simulink model "gm_uz_pmsm_model_9ph_dq"  (R2021b)
settings: Solver=FixedStepAuto  StartTime=0.0  StopTime=0.8  RelTol=1e-3
undefined symbols (not defined in the file or in its folder): c, friction_coefficient, inertia, k_i_d, k_i_q, k_p_d, k_p_q, Kpd, L_d, L_q, L_x1, L_x2, L_x3, L_y1, L_y2, L_y3, L_zero, polepair, psi_pm, R_1, static_friction_torque, Tnd
libraries: hdlmdlgenlib x137, dspsigops x19, slpidlib x2, pid_lib x1, spsdq0toAlphaBetaZeroLib x1
(part 2 of 2)

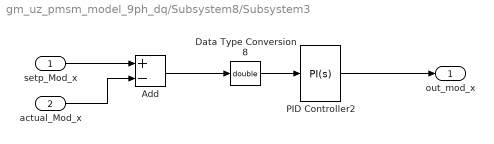
== system gm_uz_pmsm_model_9ph_dq/Subsystem8/Subsystem3 ==
  setp_Mod_x : Inport
  actual_Mod_x : Inport  Port=2
  Add : Sum  Inputs=+-
  Data Type Conversion8 : DataTypeConversion  OutDataTypeStr=double
  PID Controller2 : slpidlib/PID Controller  Controller=PI  Form=Ideal  TimeDomain=Continuous-time  UseExternalTs=off  SampleTime=-1  IntegratorMethod=Forward Euler  FilterMethod=Forward Euler  ControllerParametersSource=internal  P=k_p_q  I=k_i_q  D=0  UseFilter=on  N=100  TunerSelectOption=Transfer Function Based (PID Tuner App)  InitialConditionSource=internal  InitialConditionForIntegrator=0  InitialConditionForFilter=0  DifferentiatorICPrevScaledInput=0  ExternalReset=none  TrackingMode=off  Kt=1  LimitOutput=on  SatLimitsSource=internal  UpperSaturationLimit=100  LowerSaturationLimit=-100  LinearizeAsGain=on  AntiWindupMode=clamping  Kb=1  POutMin=[]  POutMax=[]  IOutMin=[]  IOutMax=[]  DOutMin=[]  DOutMax=[]  NOutMin=[]  NOutMax=[]  SumOutMin=[]  SumOutMax=[]  SaturationOutMin=[]  SaturationOutMax=[]  PParamMin=[]  PParamMax=[]  IParamMin=[]  IParamMax=[]  DParamMin=[]  DParamMax=[]  NParamMin=[]  NParamMax=[]  KbParamMin=[]  KbParamMax=[]  KtParamMin=[]  KtParamMax=[]  KbOutMin=[]  KbOutMax=[]  KtOutMin=[]  KtOutMax=[]  IntegratorOutMin=[]  IntegratorOutMax=[]  FilterOutMin=[]  FilterOutMax=[]  SumI1OutMin=[]  SumI1OutMax=[]  SumI2OutMin=[]  SumI2OutMax=[]  SumI3OutMin=[]  SumI3OutMax=[]  SumI4OutMin=[]  SumI4OutMax=[]  SumDOutMin=[]  SumDOutMax=[]  DifferentiatorOutMin=[]  DifferentiatorOutMax=[]  FilterDiffOutCoefMin=[]  FilterDiffOutCoefMax=[]  ReciprocalOutMin=[]  ReciprocalOutMax=[]  SumDenOutMin=[]  SumDenOutMax=[]  SumNumOutMin=[]  SumNumOutMax=[]  DivideOutMin=[]  DivideOutMax=[]  UdiffTsProdOutMin=[]  UdiffTsProdOutMax=[]  NTsProdOutMin=[]  NTsProdOutMax=[]  UintegralTsProdOutMin=[]  UintegralTsProdOutMax=[]  UngainTsProdOutMin=[]  UngainTsProdOutMax=[]  IntegratorContinuousStateAttributes=''  IntegratorStateMustResolveToSignalObject=off  IntegratorRTWStateStorageClass=Auto  FilterContinuousStateAttributes=''  FilterStateMustResolveToSignalObject=off  FilterRTWStateStorageClass=Auto  ParallelPVariant=Passthrough  IdealPVariant=InternalParameters  IVariant=InternalParameters  DVariant=Disabled  IntegratorVariant=Continuous  SatVariant=Enabled  AWVariant=ContClampingIdeal  PCopyVariant=InternalParamsIdeal  TRVariant=Disabled  FdbkBlocksVariant=Forward  IdealPFdbkVariant=Disabled  SatFdbkVariant=Disabled  DerivativeFilterVariant=Disabled  NVariant=Disabled  NCopyVariant=Disabled_SignalSpec  FilterICVariant=Disabled  IntegratorICVariant=InternalICs  ExternalResetVariant=Disabled  TRSumVariant=Passthrough  SumFdbkVariant=Disabled  SumVariant=Sum_PI  TsampFilterVariant=InternalTs  TsampNgainVariant=Passthrough  TsampIntegralVariant=Passthrough  ExternalSaturationOutDataTypeStr=Inherit: Same as second input
  out_mod_x : Outport
  wires:
  Add/1 -> Data Type Conversion8/1
  actual_Mod_x/1 -> Add/2
  Data Type Conversion8/1 -> PID Controller2/1
  setp_Mod_x/1 -> Add/1
  PID Controller2/1 -> out_mod_x/1

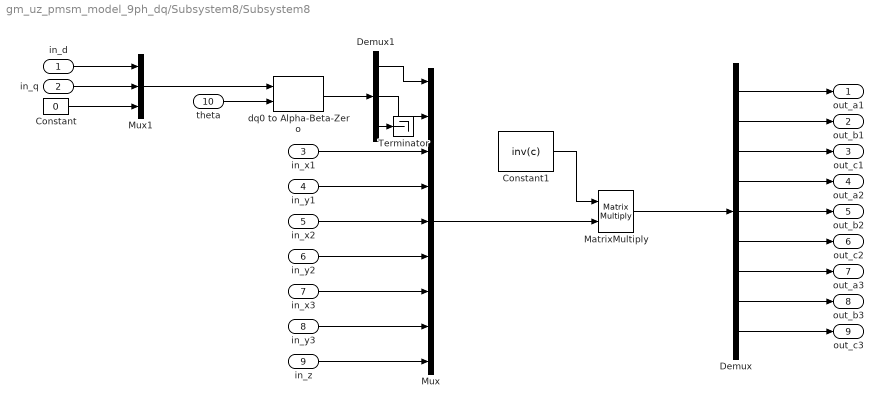
== system gm_uz_pmsm_model_9ph_dq/Subsystem8/Subsystem8 ==
  in_d : Inport
  in_q : Inport  Port=2
  in_x1 : Inport  Port=3
  in_y1 : Inport  Port=4
  in_x2 : Inport  Port=5
  in_y2 : Inport  Port=6
  in_x3 : Inport  Port=7
  in_y3 : Inport  Port=8
  in_z : Inport  Port=9
  theta : Inport  Port=10
  Constant : Constant  Value=0  SampleTime=-1
  Constant1 : Constant  Value=inv(c)
  Demux : Demux  Outputs=9
  Demux1 : Demux  Outputs=3
  MatrixMultiply : Product  Multiplication=Matrix(*)
  Mux : Mux  Inputs=9
  Mux1 : Mux  Inputs=3
  Terminator : Terminator
  dq0 to Alpha-Beta-Zero : spsdq0toAlphaBetaZeroLib/dq0 to Alpha-Beta-Zero  Alignment=90 degrees behind phase A axis
      settings: SourceProductBaseCode=PS
  out_a1 : Outport
  out_b1 : Outport  Port=2
  out_c1 : Outport  Port=3
  out_a2 : Outport  Port=4
  out_b2 : Outport  Port=5
  out_c2 : Outport  Port=6
  out_a3 : Outport  Port=7
  out_b3 : Outport  Port=8
  out_c3 : Outport  Port=9
  wires:
  Demux/7 -> out_a3/1
  Demux/9 -> out_c3/1
  Demux/8 -> out_b3/1
  Demux/5 -> out_b2/1
  Demux/6 -> out_c2/1
  Demux/4 -> out_a2/1
  Demux/3 -> out_c1/1
  Demux/2 -> out_b1/1
  Constant1/1 -> MatrixMultiply/1
  Demux1/3 -> Terminator/1
  Demux1/2 -> Mux/2
  Demux1/1 -> Mux/1
  dq0 to Alpha-Beta-Zero/1 -> Demux1/1
  theta/1 -> dq0 to Alpha-Beta-Zero/2
  Mux1/1 -> dq0 to Alpha-Beta-Zero/1
  in_d/1 -> Mux1/1
  in_q/1 -> Mux1/2
  Constant/1 -> Mux1/3
  in_z/1 -> Mux/9
  in_x2/1 -> Mux/5
  Mux/1 -> MatrixMultiply/2
  in_y1/1 -> Mux/4
  in_x1/1 -> Mux/3
  Demux/1 -> out_a1/1
  in_y2/1 -> Mux/6
  MatrixMultiply/1 -> Demux/1
  in_y3/1 -> Mux/8
  in_x3/1 -> Mux/7

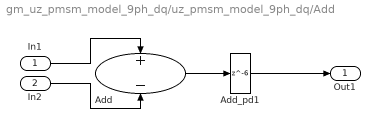
== system gm_uz_pmsm_model_9ph_dq/uz_pmsm_model_9ph_dq/Add ==
  In1 : Inport
  In2 : Inport  Port=2
  Add : Sum  Inputs=+-  OutDataTypeStr=double  SampleTime=1e-08
  Add_pd1 : Delay  DelayLength=6
  Out1 : Outport
  wires:
  In1/1 -> Add/1
  In2/1 -> Add/2
  Add/1 -> Add_pd1/1
  Add_pd1/1 -> Out1/1

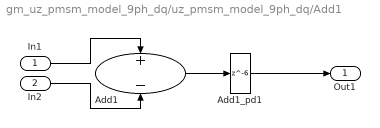
== system gm_uz_pmsm_model_9ph_dq/uz_pmsm_model_9ph_dq/Add1 ==
  In1 : Inport
  In2 : Inport  Port=2
  Add1 : Sum  Inputs=+-  OutDataTypeStr=double  SampleTime=1e-08
  Add1_pd1 : Delay  DelayLength=6
  Out1 : Outport
  wires:
  In1/1 -> Add1/1
  In2/1 -> Add1/2
  Add1/1 -> Add1_pd1/1
  Add1_pd1/1 -> Out1/1

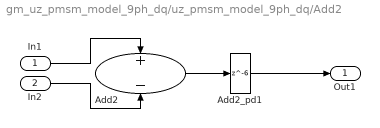
== system gm_uz_pmsm_model_9ph_dq/uz_pmsm_model_9ph_dq/Add2 ==
  In1 : Inport
  In2 : Inport  Port=2
  Add2 : Sum  Inputs=+-  OutDataTypeStr=double  SampleTime=1e-08
  Add2_pd1 : Delay  DelayLength=6
  Out1 : Outport
  wires:
  In1/1 -> Add2/1
  In2/1 -> Add2/2
  Add2/1 -> Add2_pd1/1
  Add2_pd1/1 -> Out1/1

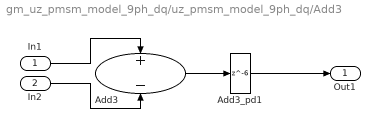
== system gm_uz_pmsm_model_9ph_dq/uz_pmsm_model_9ph_dq/Add3 ==
  In1 : Inport
  In2 : Inport  Port=2
  Add3 : Sum  Inputs=+-  OutDataTypeStr=double  SampleTime=1e-08
  Add3_pd1 : Delay  DelayLength=6
  Out1 : Outport
  wires:
  In1/1 -> Add3/1
  In2/1 -> Add3/2
  Add3/1 -> Add3_pd1/1
  Add3_pd1/1 -> Out1/1

== system gm_uz_pmsm_model_9ph_dq/uz_pmsm_model_9ph_dq/Add4 ==
  In1 : Inport
  In2 : Inport  Port=2
  Add4 : Sum  Inputs=+-  OutDataTypeStr=double  SampleTime=1e-08
  Add4_pd1 : Delay  DelayLength=6
  Out1 : Outport
  wires:
  In1/1 -> Add4/1
  In2/1 -> Add4/2
  Add4/1 -> Add4_pd1/1
  Add4_pd1/1 -> Out1/1

== system gm_uz_pmsm_model_9ph_dq/uz_pmsm_model_9ph_dq/Add5 ==
  In1 : Inport
  In2 : Inport  Port=2
  Add5 : Sum  Inputs=+-  OutDataTypeStr=double  SampleTime=1e-08
  Add5_pd1 : Delay  DelayLength=6
  Out1 : Outport
  wires:
  In1/1 -> Add5/1
  In2/1 -> Add5/2
  Add5/1 -> Add5_pd1/1
  Add5_pd1/1 -> Out1/1

== system gm_uz_pmsm_model_9ph_dq/uz_pmsm_model_9ph_dq/Add6 ==
  In1 : Inport
  In2 : Inport  Port=2
  Add6 : Sum  Inputs=+-  OutDataTypeStr=double  SampleTime=1e-08
  Add6_pd1 : Delay  DelayLength=6
  Out1 : Outport
  wires:
  In1/1 -> Add6/1
  In2/1 -> Add6/2
  Add6/1 -> Add6_pd1/1
  Add6_pd1/1 -> Out1/1

== system gm_uz_pmsm_model_9ph_dq/uz_pmsm_model_9ph_dq/Compare To Constant1_relop ==
  In1 : Inport
  In2 : Inport  Port=2
  Compare To Constant1_relop : RelationalOperator  Operator=<  OutDataTypeStr=boolean  SampleTime=1e-08  RndMeth=Nearest  InputSameDT=on
  Compare To Constant1_relop_pd1 : Delay  DelayLength=1
  Out1 : Outport
  wires:
  In1/1 -> Compare To Constant1_relop/1
  In2/1 -> Compare To Constant1_relop/2
  Compare To Constant1_relop/1 -> Compare To Constant1_relop_pd1/1
  Compare To Constant1_relop_pd1/1 -> Out1/1

== system gm_uz_pmsm_model_9ph_dq/uz_pmsm_model_9ph_dq/Compare To Constant_relop ==
  In1 : Inport
  In2 : Inport  Port=2
  Compare To Constant_relop : RelationalOperator  OutDataTypeStr=boolean  SampleTime=1e-08  RndMeth=Nearest  InputSameDT=on
  Compare To Constant_relop_pd1 : Delay  DelayLength=1
  Out1 : Outport
  wires:
  In1/1 -> Compare To Constant_relop/1
  In2/1 -> Compare To Constant_relop/2
  Compare To Constant_relop/1 -> Compare To Constant_relop_pd1/1
  Compare To Constant_relop_pd1/1 -> Out1/1

== system gm_uz_pmsm_model_9ph_dq/uz_pmsm_model_9ph_dq/Data Type Conversion1 ==
  In1 : Inport
  Data Type Conversion1 : DataTypeConversion  OutDataTypeStr=double  RndMeth=Nearest  SampleTime=1e-08
  Data Type Conversion1_pd1 : Delay  DelayLength=3
  Out1 : Outport
  wires:
  In1/1 -> Data Type Conversion1/1
  Data Type Conversion1/1 -> Data Type Conversion1_pd1/1
  Data Type Conversion1_pd1/1 -> Out1/1

== system gm_uz_pmsm_model_9ph_dq/uz_pmsm_model_9ph_dq/Data Type Conversion10 ==
  In1 : Inport
  Data Type Conversion10 : DataTypeConversion  OutDataTypeStr=double  RndMeth=Nearest  SampleTime=1e-08
  Data Type Conversion10_pd1 : Delay  DelayLength=3
  Out1 : Outport
  wires:
  In1/1 -> Data Type Conversion10/1
  Data Type Conversion10/1 -> Data Type Conversion10_pd1/1
  Data Type Conversion10_pd1/1 -> Out1/1

== system gm_uz_pmsm_model_9ph_dq/uz_pmsm_model_9ph_dq/Data Type Conversion101 ==
  In1 : Inport
  Data Type Conversion101 : DataTypeConversion  OutDataTypeStr=double  RndMeth=Nearest  SampleTime=1e-08
  Data Type Conversion101_pd1 : Delay  DelayLength=3
  Out1 : Outport
  wires:
  In1/1 -> Data Type Conversion101/1
  Data Type Conversion101/1 -> Data Type Conversion101_pd1/1
  Data Type Conversion101_pd1/1 -> Out1/1

== system gm_uz_pmsm_model_9ph_dq/uz_pmsm_model_9ph_dq/Data Type Conversion11 ==
  In1 : Inport
  Data Type Conversion11 : DataTypeConversion  OutDataTypeStr=single  RndMeth=Nearest  SampleTime=1e-08
  Data Type Conversion11_pd1 : Delay  DelayLength=3
  Out1 : Outport
  wires:
  In1/1 -> Data Type Conversion11/1
  Data Type Conversion11/1 -> Data Type Conversion11_pd1/1
  Data Type Conversion11_pd1/1 -> Out1/1

== system gm_uz_pmsm_model_9ph_dq/uz_pmsm_model_9ph_dq/Data Type Conversion111 ==
  In1 : Inport
  Data Type Conversion111 : DataTypeConversion  OutDataTypeStr=double  RndMeth=Nearest  SampleTime=1e-08
  Data Type Conversion111_pd1 : Delay  DelayLength=3
  Out1 : Outport
  wires:
  In1/1 -> Data Type Conversion111/1
  Data Type Conversion111/1 -> Data Type Conversion111_pd1/1
  Data Type Conversion111_pd1/1 -> Out1/1

== system gm_uz_pmsm_model_9ph_dq/uz_pmsm_model_9ph_dq/Data Type Conversion12 ==
  In1 : Inport
  Data Type Conversion12 : DataTypeConversion  OutDataTypeStr=fixdt(1, 18, 14)  RndMeth=Nearest  SampleTime=1e-08
  Data Type Conversion12_pd1 : Delay  DelayLength=3
  Out1 : Outport
  wires:
  In1/1 -> Data Type Conversion12/1
  Data Type Conversion12/1 -> Data Type Conversion12_pd1/1
  Data Type Conversion12_pd1/1 -> Out1/1

== system gm_uz_pmsm_model_9ph_dq/uz_pmsm_model_9ph_dq/Data Type Conversion121 ==
  In1 : Inport
  Data Type Conversion121 : DataTypeConversion  OutDataTypeStr=double  RndMeth=Nearest  SampleTime=1e-08
  Data Type Conversion121_pd1 : Delay  DelayLength=3
  Out1 : Outport
  wires:
  In1/1 -> Data Type Conversion121/1
  Data Type Conversion121/1 -> Data Type Conversion121_pd1/1
  Data Type Conversion121_pd1/1 -> Out1/1

== system gm_uz_pmsm_model_9ph_dq/uz_pmsm_model_9ph_dq/Data Type Conversion13 ==
  In1 : Inport
  Data Type Conversion13 : DataTypeConversion  OutDataTypeStr=double  RndMeth=Nearest  SampleTime=1e-08
  Data Type Conversion13_pd1 : Delay  DelayLength=3
  Out1 : Outport
  wires:
  In1/1 -> Data Type Conversion13/1
  Data Type Conversion13/1 -> Data Type Conversion13_pd1/1
  Data Type Conversion13_pd1/1 -> Out1/1

== system gm_uz_pmsm_model_9ph_dq/uz_pmsm_model_9ph_dq/Data Type Conversion14 ==
  In1 : Inport
  Data Type Conversion14 : DataTypeConversion  OutDataTypeStr=single  RndMeth=Nearest  SampleTime=1e-08
  Data Type Conversion14_pd1 : Delay  DelayLength=3
  Out1 : Outport
  wires:
  In1/1 -> Data Type Conversion14/1
  Data Type Conversion14/1 -> Data Type Conversion14_pd1/1
  Data Type Conversion14_pd1/1 -> Out1/1

== system gm_uz_pmsm_model_9ph_dq/uz_pmsm_model_9ph_dq/Data Type Conversion15 ==
  In1 : Inport
  Data Type Conversion15 : DataTypeConversion  OutDataTypeStr=double  RndMeth=Nearest  SampleTime=1e-08
  Data Type Conversion15_pd1 : Delay  DelayLength=3
  Out1 : Outport
  wires:
  In1/1 -> Data Type Conversion15/1
  Data Type Conversion15/1 -> Data Type Conversion15_pd1/1
  Data Type Conversion15_pd1/1 -> Out1/1

== system gm_uz_pmsm_model_9ph_dq/uz_pmsm_model_9ph_dq/Data Type Conversion2 ==
  In1 : Inport
  Data Type Conversion2 : DataTypeConversion  OutDataTypeStr=double  RndMeth=Nearest  SampleTime=1e-08
  Data Type Conversion2_pd1 : Delay  DelayLength=3
  Out1 : Outport
  wires:
  In1/1 -> Data Type Conversion2/1
  Data Type Conversion2/1 -> Data Type Conversion2_pd1/1
  Data Type Conversion2_pd1/1 -> Out1/1

== system gm_uz_pmsm_model_9ph_dq/uz_pmsm_model_9ph_dq/Data Type Conversion21 ==
  In1 : Inport
  Data Type Conversion21 : DataTypeConversion  OutDataTypeStr=double  RndMeth=Nearest  SampleTime=1e-08
  Data Type Conversion21_pd1 : Delay  DelayLength=3
  Out1 : Outport
  wires:
  In1/1 -> Data Type Conversion21/1
  Data Type Conversion21/1 -> Data Type Conversion21_pd1/1
  Data Type Conversion21_pd1/1 -> Out1/1

== system gm_uz_pmsm_model_9ph_dq/uz_pmsm_model_9ph_dq/Data Type Conversion3 ==
  In1 : Inport
  Data Type Conversion3 : DataTypeConversion  OutDataTypeStr=fixdt(1, 27, 18)  RndMeth=Nearest  SampleTime=1e-08
  Data Type Conversion3_pd1 : Delay  DelayLength=3
  Out1 : Outport
  wires:
  In1/1 -> Data Type Conversion3/1
  Data Type Conversion3/1 -> Data Type Conversion3_pd1/1
  Data Type Conversion3_pd1/1 -> Out1/1

== system gm_uz_pmsm_model_9ph_dq/uz_pmsm_model_9ph_dq/Data Type Conversion31 ==
  In1 : Inport
  Data Type Conversion31 : DataTypeConversion  OutDataTypeStr=double  RndMeth=Nearest  SampleTime=1e-08
  Data Type Conversion31_pd1 : Delay  DelayLength=3
  Out1 : Outport
  wires:
  In1/1 -> Data Type Conversion31/1
  Data Type Conversion31/1 -> Data Type Conversion31_pd1/1
  Data Type Conversion31_pd1/1 -> Out1/1

== system gm_uz_pmsm_model_9ph_dq/uz_pmsm_model_9ph_dq/Data Type Conversion4 ==
  In1 : Inport
  Data Type Conversion4 : DataTypeConversion  OutDataTypeStr=single  RndMeth=Nearest  SampleTime=1e-08
  Data Type Conversion4_pd1 : Delay  DelayLength=3
  Out1 : Outport
  wires:
  In1/1 -> Data Type Conversion4/1
  Data Type Conversion4/1 -> Data Type Conversion4_pd1/1
  Data Type Conversion4_pd1/1 -> Out1/1

== system gm_uz_pmsm_model_9ph_dq/uz_pmsm_model_9ph_dq/Data Type Conversion41 ==
  In1 : Inport
  Data Type Conversion41 : DataTypeConversion  OutDataTypeStr=double  RndMeth=Nearest  SampleTime=1e-08
  Data Type Conversion41_pd1 : Delay  DelayLength=3
  Out1 : Outport
  wires:
  In1/1 -> Data Type Conversion41/1
  Data Type Conversion41/1 -> Data Type Conversion41_pd1/1
  Data Type Conversion41_pd1/1 -> Out1/1

== system gm_uz_pmsm_model_9ph_dq/uz_pmsm_model_9ph_dq/Data Type Conversion5 ==
  In1 : Inport
  Data Type Conversion5 : DataTypeConversion  OutDataTypeStr=single  RndMeth=Nearest  SampleTime=1e-08
  Data Type Conversion5_pd1 : Delay  DelayLength=3
  Out1 : Outport
  wires:
  In1/1 -> Data Type Conversion5/1
  Data Type Conversion5/1 -> Data Type Conversion5_pd1/1
  Data Type Conversion5_pd1/1 -> Out1/1

== system gm_uz_pmsm_model_9ph_dq/uz_pmsm_model_9ph_dq/Data Type Conversion51 ==
  In1 : Inport
  Data Type Conversion51 : DataTypeConversion  OutDataTypeStr=double  RndMeth=Nearest  SampleTime=1e-08
  Data Type Conversion51_pd1 : Delay  DelayLength=3
  Out1 : Outport
  wires:
  In1/1 -> Data Type Conversion51/1
  Data Type Conversion51/1 -> Data Type Conversion51_pd1/1
  Data Type Conversion51_pd1/1 -> Out1/1

== system gm_uz_pmsm_model_9ph_dq/uz_pmsm_model_9ph_dq/Data Type Conversion6 ==
  In1 : Inport
  Data Type Conversion6 : DataTypeConversion  OutDataTypeStr=double  RndMeth=Nearest  SampleTime=1e-08
  Data Type Conversion6_pd1 : Delay  DelayLength=3
  Out1 : Outport
  wires:
  In1/1 -> Data Type Conversion6/1
  Data Type Conversion6/1 -> Data Type Conversion6_pd1/1
  Data Type Conversion6_pd1/1 -> Out1/1

== system gm_uz_pmsm_model_9ph_dq/uz_pmsm_model_9ph_dq/Data Type Conversion61 ==
  In1 : Inport
  Data Type Conversion61 : DataTypeConversion  OutDataTypeStr=double  RndMeth=Nearest  SampleTime=1e-08
  Data Type Conversion61_pd1 : Delay  DelayLength=3
  Out1 : Outport
  wires:
  In1/1 -> Data Type Conversion61/1
  Data Type Conversion61/1 -> Data Type Conversion61_pd1/1
  Data Type Conversion61_pd1/1 -> Out1/1

== system gm_uz_pmsm_model_9ph_dq/uz_pmsm_model_9ph_dq/Data Type Conversion7 ==
  In1 : Inport
  Data Type Conversion7 : DataTypeConversion  OutDataTypeStr=double  RndMeth=Nearest  SampleTime=1e-08
  Data Type Conversion7_pd1 : Delay  DelayLength=3
  Out1 : Outport
  wires:
  In1/1 -> Data Type Conversion7/1
  Data Type Conversion7/1 -> Data Type Conversion7_pd1/1
  Data Type Conversion7_pd1/1 -> Out1/1

== system gm_uz_pmsm_model_9ph_dq/uz_pmsm_model_9ph_dq/Data Type Conversion71 ==
  In1 : Inport
  Data Type Conversion71 : DataTypeConversion  OutDataTypeStr=double  RndMeth=Nearest  SampleTime=1e-08
  Data Type Conversion71_pd1 : Delay  DelayLength=3
  Out1 : Outport
  wires:
  In1/1 -> Data Type Conversion71/1
  Data Type Conversion71/1 -> Data Type Conversion71_pd1/1
  Data Type Conversion71_pd1/1 -> Out1/1

== system gm_uz_pmsm_model_9ph_dq/uz_pmsm_model_9ph_dq/Data Type Conversion8 ==
  In1 : Inport
  Data Type Conversion8 : DataTypeConversion  OutDataTypeStr=double  RndMeth=Nearest  SampleTime=1e-08
  Data Type Conversion8_pd1 : Delay  DelayLength=3
  Out1 : Outport
  wires:
  In1/1 -> Data Type Conversion8/1
  Data Type Conversion8/1 -> Data Type Conversion8_pd1/1
  Data Type Conversion8_pd1/1 -> Out1/1

== system gm_uz_pmsm_model_9ph_dq/uz_pmsm_model_9ph_dq/Data Type Conversion81 ==
  In1 : Inport
  Data Type Conversion81 : DataTypeConversion  OutDataTypeStr=single  RndMeth=Nearest  SampleTime=1e-08
  Data Type Conversion81_pd1 : Delay  DelayLength=3
  Out1 : Outport
  wires:
  In1/1 -> Data Type Conversion81/1
  Data Type Conversion81/1 -> Data Type Conversion81_pd1/1
  Data Type Conversion81_pd1/1 -> Out1/1

== system gm_uz_pmsm_model_9ph_dq/uz_pmsm_model_9ph_dq/Data Type Conversion9 ==
  In1 : Inport
  Data Type Conversion9 : DataTypeConversion  OutDataTypeStr=double  RndMeth=Nearest  SampleTime=1e-08
  Data Type Conversion9_pd1 : Delay  DelayLength=3
  Out1 : Outport
  wires:
  In1/1 -> Data Type Conversion9/1
  Data Type Conversion9/1 -> Data Type Conversion9_pd1/1
  Data Type Conversion9_pd1/1 -> Out1/1

== system gm_uz_pmsm_model_9ph_dq/uz_pmsm_model_9ph_dq/Divide ==
  In1 : Inport
  In2 : Inport  Port=2
  Divide : Product  Inputs=**  OutDataTypeStr=double  SampleTime=1e-08
  Divide_pd1 : Delay  DelayLength=6
  Out1 : Outport
  wires:
  In1/1 -> Divide/1
  In2/1 -> Divide/2
  Divide/1 -> Divide_pd1/1
  Divide_pd1/1 -> Out1/1

== system gm_uz_pmsm_model_9ph_dq/uz_pmsm_model_9ph_dq/Divide1 ==
  In1 : Inport
  In2 : Inport  Port=2
  Divide1 : Product  Inputs=**  OutDataTypeStr=double  SampleTime=1e-08
  Divide1_pd1 : Delay  DelayLength=6
  Out1 : Outport
  wires:
  In1/1 -> Divide1/1
  In2/1 -> Divide1/2
  Divide1/1 -> Divide1_pd1/1
  Divide1_pd1/1 -> Out1/1

== system gm_uz_pmsm_model_9ph_dq/uz_pmsm_model_9ph_dq/Divide10 ==
  In1 : Inport
  In2 : Inport  Port=2
  Divide10 : Product  Inputs=**  OutDataTypeStr=double  SampleTime=1e-08
  Divide10_pd1 : Delay  DelayLength=6
  Out1 : Outport
  wires:
  In1/1 -> Divide10/1
  In2/1 -> Divide10/2
  Divide10/1 -> Divide10_pd1/1
  Divide10_pd1/1 -> Out1/1

== system gm_uz_pmsm_model_9ph_dq/uz_pmsm_model_9ph_dq/Divide11 ==
  In1 : Inport
  In2 : Inport  Port=2
  Divide11 : Product  Inputs=**  OutDataTypeStr=double  SampleTime=1e-08
  Divide11_pd1 : Delay  DelayLength=6
  Out1 : Outport
  wires:
  In1/1 -> Divide11/1
  In2/1 -> Divide11/2
  Divide11/1 -> Divide11_pd1/1
  Divide11_pd1/1 -> Out1/1

== system gm_uz_pmsm_model_9ph_dq/uz_pmsm_model_9ph_dq/Divide12 ==
  In1 : Inport
  In2 : Inport  Port=2
  Divide12 : Product  Inputs=**  OutDataTypeStr=double  SampleTime=1e-08
  Divide12_pd1 : Delay  DelayLength=6
  Out1 : Outport
  wires:
  In1/1 -> Divide12/1
  In2/1 -> Divide12/2
  Divide12/1 -> Divide12_pd1/1
  Divide12_pd1/1 -> Out1/1

== system gm_uz_pmsm_model_9ph_dq/uz_pmsm_model_9ph_dq/Divide13 ==
  In1 : Inport
  In2 : Inport  Port=2
  Divide13 : Product  Inputs=**  OutDataTypeStr=double  SampleTime=1e-08
  Divide13_pd1 : Delay  DelayLength=6
  Out1 : Outport
  wires:
  In1/1 -> Divide13/1
  In2/1 -> Divide13/2
  Divide13/1 -> Divide13_pd1/1
  Divide13_pd1/1 -> Out1/1

== system gm_uz_pmsm_model_9ph_dq/uz_pmsm_model_9ph_dq/Divide2 ==
  In1 : Inport
  In2 : Inport  Port=2
  Divide2 : Product  Inputs=**  OutDataTypeStr=double  SampleTime=1e-08
  Divide2_pd1 : Delay  DelayLength=6
  Out1 : Outport
  wires:
  In1/1 -> Divide2/1
  In2/1 -> Divide2/2
  Divide2/1 -> Divide2_pd1/1
  Divide2_pd1/1 -> Out1/1

== system gm_uz_pmsm_model_9ph_dq/uz_pmsm_model_9ph_dq/Divide3 ==
  In1 : Inport
  In2 : Inport  Port=2
  Divide3 : Product  Inputs=**  OutDataTypeStr=double  SampleTime=1e-08
  Divide3_pd1 : Delay  DelayLength=6
  Out1 : Outport
  wires:
  In1/1 -> Divide3/1
  In2/1 -> Divide3/2
  Divide3/1 -> Divide3_pd1/1
  Divide3_pd1/1 -> Out1/1

== system gm_uz_pmsm_model_9ph_dq/uz_pmsm_model_9ph_dq/Divide4 ==
  In1 : Inport
  In2 : Inport  Port=2
  Divide4 : Product  Inputs=**  OutDataTypeStr=double  SampleTime=1e-08
  Divide4_pd1 : Delay  DelayLength=6
  Out1 : Outport
  wires:
  In1/1 -> Divide4/1
  In2/1 -> Divide4/2
  Divide4/1 -> Divide4_pd1/1
  Divide4_pd1/1 -> Out1/1

== system gm_uz_pmsm_model_9ph_dq/uz_pmsm_model_9ph_dq/Divide5 ==
  In1 : Inport
  In2 : Inport  Port=2
  Divide5 : Product  Inputs=**  OutDataTypeStr=double  SampleTime=1e-08
  Divide5_pd1 : Delay  DelayLength=6
  Out1 : Outport
  wires:
  In1/1 -> Divide5/1
  In2/1 -> Divide5/2
  Divide5/1 -> Divide5_pd1/1
  Divide5_pd1/1 -> Out1/1

== system gm_uz_pmsm_model_9ph_dq/uz_pmsm_model_9ph_dq/Divide6 ==
  In1 : Inport
  In2 : Inport  Port=2
  Divide6 : Product  Inputs=**  OutDataTypeStr=double  SampleTime=1e-08
  Divide6_pd1 : Delay  DelayLength=6
  Out1 : Outport
  wires:
  In1/1 -> Divide6/1
  In2/1 -> Divide6/2
  Divide6/1 -> Divide6_pd1/1
  Divide6_pd1/1 -> Out1/1

== system gm_uz_pmsm_model_9ph_dq/uz_pmsm_model_9ph_dq/Divide7 ==
  In1 : Inport
  In2 : Inport  Port=2
  Divide7 : Product  Inputs=**  OutDataTypeStr=double  SampleTime=1e-08
  Divide7_pd1 : Delay  DelayLength=6
  Out1 : Outport
  wires:
  In1/1 -> Divide7/1
  In2/1 -> Divide7/2
  Divide7/1 -> Divide7_pd1/1
  Divide7_pd1/1 -> Out1/1

== system gm_uz_pmsm_model_9ph_dq/uz_pmsm_model_9ph_dq/Divide8 ==
  In1 : Inport
  In2 : Inport  Port=2
  Divide8 : Product  Inputs=**  OutDataTypeStr=double  SampleTime=1e-08
  Divide8_pd1 : Delay  DelayLength=6
  Out1 : Outport
  wires:
  In1/1 -> Divide8/1
  In2/1 -> Divide8/2
  Divide8/1 -> Divide8_pd1/1
  Divide8_pd1/1 -> Out1/1

== system gm_uz_pmsm_model_9ph_dq/uz_pmsm_model_9ph_dq/Divide9 ==
  In1 : Inport
  In2 : Inport  Port=2
  Divide9 : Product  Inputs=**  OutDataTypeStr=double  SampleTime=1e-08
  Divide9_pd1 : Delay  DelayLength=6
  Out1 : Outport
  wires:
  In1/1 -> Divide9/1
  In2/1 -> Divide9/2
  Divide9/1 -> Divide9_pd1/1
  Divide9_pd1/1 -> Out1/1

== system gm_uz_pmsm_model_9ph_dq/uz_pmsm_model_9ph_dq/Factor ==
  In1 : Inport
  In2 : Inport  Port=2
  Factor : Product  Inputs=**  OutDataTypeStr=double  SampleTime=1e-08
  Factor_pd1 : Delay  DelayLength=6
  Out1 : Outport
  wires:
  In1/1 -> Factor/1
  In2/1 -> Factor/2
  Factor/1 -> Factor_pd1/1
  Factor_pd1/1 -> Out1/1

== system gm_uz_pmsm_model_9ph_dq/uz_pmsm_model_9ph_dq/Gain ==
  In1 : Inport
  In2 : Inport  Port=2
  Gain : Product  Inputs=**  OutDataTypeStr=double  SampleTime=1e-08
  Gain_pd1 : Delay  DelayLength=6
  Out1 : Outport
  wires:
  In1/1 -> Gain/1
  In2/1 -> Gain/2
  Gain/1 -> Gain_pd1/1
  Gain_pd1/1 -> Out1/1

== system gm_uz_pmsm_model_9ph_dq/uz_pmsm_model_9ph_dq/Gain1 ==
  In1 : Inport
  In2 : Inport  Port=2
  Gain1 : Product  Inputs=**  OutDataTypeStr=double  SampleTime=1e-08
  Gain1_pd1 : Delay  DelayLength=6
  Out1 : Outport
  wires:
  In1/1 -> Gain1/1
  In2/1 -> Gain1/2
  Gain1/1 -> Gain1_pd1/1
  Gain1_pd1/1 -> Out1/1

== system gm_uz_pmsm_model_9ph_dq/uz_pmsm_model_9ph_dq/Gain10 ==
  In1 : Inport
  In2 : Inport  Port=2
  Gain10 : Product  Inputs=**  OutDataTypeStr=double  SampleTime=1e-08
  Gain10_pd1 : Delay  DelayLength=6
  Out1 : Outport
  wires:
  In1/1 -> Gain10/1
  In2/1 -> Gain10/2
  Gain10/1 -> Gain10_pd1/1
  Gain10_pd1/1 -> Out1/1

== system gm_uz_pmsm_model_9ph_dq/uz_pmsm_model_9ph_dq/Gain2 ==
  In1 : Inport
  In2 : Inport  Port=2
  Gain2 : Product  Inputs=**  OutDataTypeStr=double  SampleTime=1e-08
  Gain2_pd1 : Delay  DelayLength=6
  Out1 : Outport
  wires:
  In1/1 -> Gain2/1
  In2/1 -> Gain2/2
  Gain2/1 -> Gain2_pd1/1
  Gain2_pd1/1 -> Out1/1

== system gm_uz_pmsm_model_9ph_dq/uz_pmsm_model_9ph_dq/Gain3 ==
  In1 : Inport
  In2 : Inport  Port=2
  Gain3 : Product  Inputs=**  OutDataTypeStr=double  SampleTime=1e-08
  Gain3_pd1 : Delay  DelayLength=6
  Out1 : Outport
  wires:
  In1/1 -> Gain3/1
  In2/1 -> Gain3/2
  Gain3/1 -> Gain3_pd1/1
  Gain3_pd1/1 -> Out1/1

== system gm_uz_pmsm_model_9ph_dq/uz_pmsm_model_9ph_dq/Gain4 ==
  In1 : Inport
  In2 : Inport  Port=2
  Gain4 : Product  Inputs=**  OutDataTypeStr=double  SampleTime=1e-08
  Gain4_pd1 : Delay  DelayLength=6
  Out1 : Outport
  wires:
  In1/1 -> Gain4/1
  In2/1 -> Gain4/2
  Gain4/1 -> Gain4_pd1/1
  Gain4_pd1/1 -> Out1/1

== system gm_uz_pmsm_model_9ph_dq/uz_pmsm_model_9ph_dq/Gain5 ==
  In1 : Inport
  In2 : Inport  Port=2
  Gain5 : Product  Inputs=**  OutDataTypeStr=double  SampleTime=1e-08
  Gain5_pd1 : Delay  DelayLength=6
  Out1 : Outport
  wires:
  In1/1 -> Gain5/1
  In2/1 -> Gain5/2
  Gain5/1 -> Gain5_pd1/1
  Gain5_pd1/1 -> Out1/1

== system gm_uz_pmsm_model_9ph_dq/uz_pmsm_model_9ph_dq/Gain6 ==
  In1 : Inport
  In2 : Inport  Port=2
  Gain6 : Product  Inputs=**  OutDataTypeStr=double  SampleTime=1e-08
  Gain6_pd1 : Delay  DelayLength=6
  Out1 : Outport
  wires:
  In1/1 -> Gain6/1
  In2/1 -> Gain6/2
  Gain6/1 -> Gain6_pd1/1
  Gain6_pd1/1 -> Out1/1

== system gm_uz_pmsm_model_9ph_dq/uz_pmsm_model_9ph_dq/Gain7 ==
  In1 : Inport
  In2 : Inport  Port=2
  Gain7 : Product  Inputs=**  OutDataTypeStr=double  SampleTime=1e-08
  Gain7_pd1 : Delay  DelayLength=6
  Out1 : Outport
  wires:
  In1/1 -> Gain7/1
  In2/1 -> Gain7/2
  Gain7/1 -> Gain7_pd1/1
  Gain7_pd1/1 -> Out1/1

== system gm_uz_pmsm_model_9ph_dq/uz_pmsm_model_9ph_dq/Gain8 ==
  In1 : Inport
  In2 : Inport  Port=2
  Gain8 : Product  Inputs=**  OutDataTypeStr=double  SampleTime=1e-08
  Gain8_pd1 : Delay  DelayLength=6
  Out1 : Outport
  wires:
  In1/1 -> Gain8/1
  In2/1 -> Gain8/2
  Gain8/1 -> Gain8_pd1/1
  Gain8_pd1/1 -> Out1/1

== system gm_uz_pmsm_model_9ph_dq/uz_pmsm_model_9ph_dq/Gain9 ==
  In1 : Inport
  In2 : Inport  Port=2
  Gain9 : Product  Inputs=**  OutDataTypeStr=double  SampleTime=1e-08
  Gain9_pd1 : Delay  DelayLength=6
  Out1 : Outport
  wires:
  In1/1 -> Gain9/1
  In2/1 -> Gain9/2
  Gain9/1 -> Gain9_pd1/1
  Gain9_pd1/1 -> Out1/1

== system gm_uz_pmsm_model_9ph_dq/uz_pmsm_model_9ph_dq/Product ==
  In1 : Inport
  In2 : Inport  Port=2
  Product : Product  Inputs=**  OutDataTypeStr=double  SampleTime=1e-08
  Product_pd1 : Delay  DelayLength=6
  Out1 : Outport
  wires:
  In1/1 -> Product/1
  In2/1 -> Product/2
  Product/1 -> Product_pd1/1
  Product_pd1/1 -> Out1/1

== system gm_uz_pmsm_model_9ph_dq/uz_pmsm_model_9ph_dq/Product1 ==
  In1 : Inport
  In2 : Inport  Port=2
  Product1 : Product  Inputs=**  OutDataTypeStr=double  SampleTime=1e-08
  Product1_pd1 : Delay  DelayLength=6
  Out1 : Outport
  wires:
  In1/1 -> Product1/1
  In2/1 -> Product1/2
  Product1/1 -> Product1_pd1/1
  Product1_pd1/1 -> Out1/1

== system gm_uz_pmsm_model_9ph_dq/uz_pmsm_model_9ph_dq/Product10 ==
  In1 : Inport
  In2 : Inport  Port=2
  Product10 : Product  Inputs=**  OutDataTypeStr=double  SampleTime=1e-08
  Product10_pd1 : Delay  DelayLength=6
  Out1 : Outport
  wires:
  In1/1 -> Product10/1
  In2/1 -> Product10/2
  Product10/1 -> Product10_pd1/1
  Product10_pd1/1 -> Out1/1

== system gm_uz_pmsm_model_9ph_dq/uz_pmsm_model_9ph_dq/Product11 ==
  In1 : Inport
  In2 : Inport  Port=2
  Product11 : Product  Inputs=**  OutDataTypeStr=double  SampleTime=1e-08
  Product11_pd1 : Delay  DelayLength=6
  Out1 : Outport
  wires:
  In1/1 -> Product11/1
  In2/1 -> Product11/2
  Product11/1 -> Product11_pd1/1
  Product11_pd1/1 -> Out1/1

== system gm_uz_pmsm_model_9ph_dq/uz_pmsm_model_9ph_dq/Product2 ==
  In1 : Inport
  In2 : Inport  Port=2
  Product2 : Product  Inputs=**  OutDataTypeStr=double  SampleTime=1e-08
  Product2_pd1 : Delay  DelayLength=6
  Out1 : Outport
  wires:
  In1/1 -> Product2/1
  In2/1 -> Product2/2
  Product2/1 -> Product2_pd1/1
  Product2_pd1/1 -> Out1/1

== system gm_uz_pmsm_model_9ph_dq/uz_pmsm_model_9ph_dq/Product21 ==
  In1 : Inport
  In2 : Inport  Port=2
  Product21 : Product  Inputs=**  OutDataTypeStr=double  SampleTime=1e-08
  Product21_pd1 : Delay  DelayLength=6
  Out1 : Outport
  wires:
  In1/1 -> Product21/1
  In2/1 -> Product21/2
  Product21/1 -> Product21_pd1/1
  Product21_pd1/1 -> Out1/1

== system gm_uz_pmsm_model_9ph_dq/uz_pmsm_model_9ph_dq/Product3 ==
  In1 : Inport
  In2 : Inport  Port=2
  Product3 : Product  Inputs=**  OutDataTypeStr=double  SampleTime=1e-08
  Product3_pd1 : Delay  DelayLength=6
  Out1 : Outport
  wires:
  In1/1 -> Product3/1
  In2/1 -> Product3/2
  Product3/1 -> Product3_pd1/1
  Product3_pd1/1 -> Out1/1

== system gm_uz_pmsm_model_9ph_dq/uz_pmsm_model_9ph_dq/Product5 ==
  In1 : Inport
  In2 : Inport  Port=2
  Product5 : Product  Inputs=**  OutDataTypeStr=double  SampleTime=1e-08
  Product5_pd1 : Delay  DelayLength=6
  Out1 : Outport
  wires:
  In1/1 -> Product5/1
  In2/1 -> Product5/2
  Product5/1 -> Product5_pd1/1
  Product5_pd1/1 -> Out1/1

== system gm_uz_pmsm_model_9ph_dq/uz_pmsm_model_9ph_dq/Product6 ==
  In1 : Inport
  In2 : Inport  Port=2
  Product6 : Product  Inputs=**  OutDataTypeStr=double  SampleTime=1e-08
  Product6_pd1 : Delay  DelayLength=6
  Out1 : Outport
  wires:
  In1/1 -> Product6/1
  In2/1 -> Product6/2
  Product6/1 -> Product6_pd1/1
  Product6_pd1/1 -> Out1/1

== system gm_uz_pmsm_model_9ph_dq/uz_pmsm_model_9ph_dq/Product7 ==
  In1 : Inport
  In2 : Inport  Port=2
  Product7 : Product  Inputs=**  OutDataTypeStr=double  SampleTime=1e-08
  Product7_pd1 : Delay  DelayLength=6
  Out1 : Outport
  wires:
  In1/1 -> Product7/1
  In2/1 -> Product7/2
  Product7/1 -> Product7_pd1/1
  Product7_pd1/1 -> Out1/1

== system gm_uz_pmsm_model_9ph_dq/uz_pmsm_model_9ph_dq/Product8 ==
  In1 : Inport
  In2 : Inport  Port=2
  Product8 : Product  Inputs=**  OutDataTypeStr=double  SampleTime=1e-08
  Product8_pd1 : Delay  DelayLength=6
  Out1 : Outport
  wires:
  In1/1 -> Product8/1
  In2/1 -> Product8/2
  Product8/1 -> Product8_pd1/1
  Product8_pd1/1 -> Out1/1

== system gm_uz_pmsm_model_9ph_dq/uz_pmsm_model_9ph_dq/Product9 ==
  In1 : Inport
  In2 : Inport  Port=2
  Product9 : Product  Inputs=**  OutDataTypeStr=double  SampleTime=1e-08
  Product9_pd1 : Delay  DelayLength=6
  Out1 : Outport
  wires:
  In1/1 -> Product9/1
  In2/1 -> Product9/2
  Product9/1 -> Product9_pd1/1
  Product9_pd1/1 -> Out1/1

== system gm_uz_pmsm_model_9ph_dq/uz_pmsm_model_9ph_dq/Sum ==
  In1 : Inport
  In2 : Inport  Port=2
  Sum : Sum  OutDataTypeStr=double  SampleTime=1e-08
  Sum_pd1 : Delay  DelayLength=6
  Out1 : Outport
  wires:
  In1/1 -> Sum/1
  In2/1 -> Sum/2
  Sum/1 -> Sum_pd1/1
  Sum_pd1/1 -> Out1/1

== system gm_uz_pmsm_model_9ph_dq/uz_pmsm_model_9ph_dq/Sum1 ==
  In1 : Inport
  In2 : Inport  Port=2
  Sum1 : Sum  OutDataTypeStr=double  SampleTime=1e-08
  Sum1_pd1 : Delay  DelayLength=6
  Out1 : Outport
  wires:
  In1/1 -> Sum1/1
  In2/1 -> Sum1/2
  Sum1/1 -> Sum1_pd1/1
  Sum1_pd1/1 -> Out1/1

== system gm_uz_pmsm_model_9ph_dq/uz_pmsm_model_9ph_dq/Sum11 ==
  In1 : Inport
  In2 : Inport  Port=2
  Sum11 : Sum  Inputs=+-  OutDataTypeStr=double  SampleTime=1e-08
  Sum11_pd1 : Delay  DelayLength=6
  Out1 : Outport
  wires:
  In1/1 -> Sum11/1
  In2/1 -> Sum11/2
  Sum11/1 -> Sum11_pd1/1
  Sum11_pd1/1 -> Out1/1

== system gm_uz_pmsm_model_9ph_dq/uz_pmsm_model_9ph_dq/Sum1_stage2 ==
  In1 : Inport
  In2 : Inport  Port=2
  Sum1_stage2 : Sum  Inputs=+-  OutDataTypeStr=double  SampleTime=1e-08
  Sum1_stage2_pd1 : Delay  DelayLength=6
  Out1 : Outport
  wires:
  In1/1 -> Sum1_stage2/1
  In2/1 -> Sum1_stage2/2
  Sum1_stage2/1 -> Sum1_stage2_pd1/1
  Sum1_stage2_pd1/1 -> Out1/1

== system gm_uz_pmsm_model_9ph_dq/uz_pmsm_model_9ph_dq/Sum1_stage3 ==
  In1 : Inport
  In2 : Inport  Port=2
  Sum1_stage3 : Sum  Inputs=+-  OutDataTypeStr=double  SampleTime=1e-08
  Sum1_stage3_pd1 : Delay  DelayLength=6
  Out1 : Outport
  wires:
  In1/1 -> Sum1_stage3/1
  In2/1 -> Sum1_stage3/2
  Sum1_stage3/1 -> Sum1_stage3_pd1/1
  Sum1_stage3_pd1/1 -> Out1/1

== system gm_uz_pmsm_model_9ph_dq/uz_pmsm_model_9ph_dq/Sum2 ==
  In1 : Inport
  In2 : Inport  Port=2
  Sum2 : Sum  OutDataTypeStr=double  SampleTime=1e-08
  Sum2_pd1 : Delay  DelayLength=6
  Out1 : Outport
  wires:
  In1/1 -> Sum2/1
  In2/1 -> Sum2/2
  Sum2/1 -> Sum2_pd1/1
  Sum2_pd1/1 -> Out1/1

== system gm_uz_pmsm_model_9ph_dq/uz_pmsm_model_9ph_dq/Sum21 ==
  In1 : Inport
  In2 : Inport  Port=2
  Sum21 : Sum  Inputs=+-  OutDataTypeStr=double  SampleTime=1e-08
  Sum21_pd1 : Delay  DelayLength=6
  Out1 : Outport
  wires:
  In1/1 -> Sum21/1
  In2/1 -> Sum21/2
  Sum21/1 -> Sum21_pd1/1
  Sum21_pd1/1 -> Out1/1

== system gm_uz_pmsm_model_9ph_dq/uz_pmsm_model_9ph_dq/Sum3 ==
  In1 : Inport
  In2 : Inport  Port=2
  Sum3 : Sum  OutDataTypeStr=double  SampleTime=1e-08
  Sum3_pd1 : Delay  DelayLength=6
  Out1 : Outport
  wires:
  In1/1 -> Sum3/1
  In2/1 -> Sum3/2
  Sum3/1 -> Sum3_pd1/1
  Sum3_pd1/1 -> Out1/1

== system gm_uz_pmsm_model_9ph_dq/uz_pmsm_model_9ph_dq/Sum31 ==
  In1 : Inport
  In2 : Inport  Port=2
  Sum31 : Sum  OutDataTypeStr=double  SampleTime=1e-08
  Sum31_pd1 : Delay  DelayLength=6
  Out1 : Outport
  wires:
  In1/1 -> Sum31/1
  In2/1 -> Sum31/2
  Sum31/1 -> Sum31_pd1/1
  Sum31_pd1/1 -> Out1/1

== system gm_uz_pmsm_model_9ph_dq/uz_pmsm_model_9ph_dq/Sum310 ==
  In1 : Inport
  In2 : Inport  Port=2
  Sum310 : Sum  Inputs=+-  OutDataTypeStr=double  SampleTime=1e-08
  Sum310_pd1 : Delay  DelayLength=6
  Out1 : Outport
  wires:
  In1/1 -> Sum310/1
  In2/1 -> Sum310/2
  Sum310/1 -> Sum310_pd1/1
  Sum310_pd1/1 -> Out1/1

== system gm_uz_pmsm_model_9ph_dq/uz_pmsm_model_9ph_dq/Sum32 ==
  In1 : Inport
  In2 : Inport  Port=2
  Sum32 : Sum  OutDataTypeStr=double  SampleTime=1e-08
  Sum32_pd1 : Delay  DelayLength=6
  Out1 : Outport
  wires:
  In1/1 -> Sum32/1
  In2/1 -> Sum32/2
  Sum32/1 -> Sum32_pd1/1
  Sum32_pd1/1 -> Out1/1

== system gm_uz_pmsm_model_9ph_dq/uz_pmsm_model_9ph_dq/Sum33 ==
  In1 : Inport
  In2 : Inport  Port=2
  Sum33 : Sum  OutDataTypeStr=double  SampleTime=1e-08
  Sum33_pd1 : Delay  DelayLength=6
  Out1 : Outport
  wires:
  In1/1 -> Sum33/1
  In2/1 -> Sum33/2
  Sum33/1 -> Sum33_pd1/1
  Sum33_pd1/1 -> Out1/1

== system gm_uz_pmsm_model_9ph_dq/uz_pmsm_model_9ph_dq/Sum34 ==
  In1 : Inport
  In2 : Inport  Port=2
  Sum34 : Sum  OutDataTypeStr=double  SampleTime=1e-08
  Sum34_pd1 : Delay  DelayLength=6
  Out1 : Outport
  wires:
  In1/1 -> Sum34/1
  In2/1 -> Sum34/2
  Sum34/1 -> Sum34_pd1/1
  Sum34_pd1/1 -> Out1/1

== system gm_uz_pmsm_model_9ph_dq/uz_pmsm_model_9ph_dq/Sum35 ==
  In1 : Inport
  In2 : Inport  Port=2
  Sum35 : Sum  OutDataTypeStr=double  SampleTime=1e-08
  Sum35_pd1 : Delay  DelayLength=6
  Out1 : Outport
  wires:
  In1/1 -> Sum35/1
  In2/1 -> Sum35/2
  Sum35/1 -> Sum35_pd1/1
  Sum35_pd1/1 -> Out1/1

== system gm_uz_pmsm_model_9ph_dq/uz_pmsm_model_9ph_dq/Sum36 ==
  In1 : Inport
  In2 : Inport  Port=2
  Sum36 : Sum  OutDataTypeStr=double  SampleTime=1e-08
  Sum36_pd1 : Delay  DelayLength=6
  Out1 : Outport
  wires:
  In1/1 -> Sum36/1
  In2/1 -> Sum36/2
  Sum36/1 -> Sum36_pd1/1
  Sum36_pd1/1 -> Out1/1

== system gm_uz_pmsm_model_9ph_dq/uz_pmsm_model_9ph_dq/Sum37 ==
  In1 : Inport
  In2 : Inport  Port=2
  Sum37 : Sum  OutDataTypeStr=double  SampleTime=1e-08
  Sum37_pd1 : Delay  DelayLength=6
  Out1 : Outport
  wires:
  In1/1 -> Sum37/1
  In2/1 -> Sum37/2
  Sum37/1 -> Sum37_pd1/1
  Sum37_pd1/1 -> Out1/1

== system gm_uz_pmsm_model_9ph_dq/uz_pmsm_model_9ph_dq/Sum38 ==
  In1 : Inport
  In2 : Inport  Port=2
  Sum38 : Sum  OutDataTypeStr=double  SampleTime=1e-08
  Sum38_pd1 : Delay  DelayLength=6
  Out1 : Outport
  wires:
  In1/1 -> Sum38/1
  In2/1 -> Sum38/2
  Sum38/1 -> Sum38_pd1/1
  Sum38_pd1/1 -> Out1/1

== system gm_uz_pmsm_model_9ph_dq/uz_pmsm_model_9ph_dq/Sum39 ==
  In1 : Inport
  In2 : Inport  Port=2
  Sum39 : Sum  OutDataTypeStr=double  SampleTime=1e-08
  Sum39_pd1 : Delay  DelayLength=6
  Out1 : Outport
  wires:
  In1/1 -> Sum39/1
  In2/1 -> Sum39/2
  Sum39/1 -> Sum39_pd1/1
  Sum39_pd1/1 -> Out1/1

== system gm_uz_pmsm_model_9ph_dq/uz_pmsm_model_9ph_dq/Sum_stage2 ==
  In1 : Inport
  In2 : Inport  Port=2
  Sum_stage2 : Sum  Inputs=+-  OutDataTypeStr=double  SampleTime=1e-08
  Sum_stage2_pd1 : Delay  DelayLength=6
  Out1 : Outport
  wires:
  In1/1 -> Sum_stage2/1
  In2/1 -> Sum_stage2/2
  Sum_stage2/1 -> Sum_stage2_pd1/1
  Sum_stage2_pd1/1 -> Out1/1

== system gm_uz_pmsm_model_9ph_dq/uz_pmsm_model_9ph_dq/Sum_stage3 ==
  In1 : Inport
  In2 : Inport  Port=2
  Sum_stage3 : Sum  OutDataTypeStr=double  SampleTime=1e-08
  Sum_stage3_pd1 : Delay  DelayLength=6
  Out1 : Outport
  wires:
  In1/1 -> Sum_stage3/1
  In2/1 -> Sum_stage3/2
  Sum_stage3/1 -> Sum_stage3_pd1/1
  Sum_stage3_pd1/1 -> Out1/1
